simulink model "CartPendsys_continous"  (R2022a)
settings: Solver=VariableStepAuto  StartTime=0.0  StopTime=15  RelTol=1e-3
values from neighbouring files (symbols this model uses):
  Kr = lqr(sysC.A,sysC.B,Q,R)    [sim_pendcart.m]
  Mscale = [eye(4); zeros(2,4)]    [sim_pendcart.m]
  Mscale1 = [eye(3), eye(3)]    [sim_pendcart.m]
  Mscale2 = [eye(2), eye(2)]    [sim_pendcart.m]
  sysC = ss(A,BF,C,[0 0 0 0 0 Vn])    [sim_pendcart.m]
  sysKf = ss(A-Kf*C, [B Kf], eye(4), 0*[B Kf])    [sim_pendcart.m]
  x0 = [1.5 0 pi 0]    [sim_pendcart.m]
settings Model: Creator=samrudh.untgodpr  LastModifiedBy=samrudh.untgodpr
settings DebuggingCC: UnconnectedInputMsg=warning  UnconnectedOutputMsg=warning  UnconnectedLineMsg=warning
settings RTWCC: DLArmComputeVersion=19.05

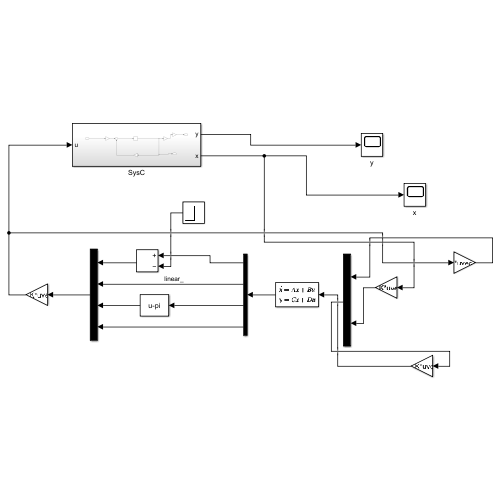
[thumbnail: Simulink's stored preview of the top-level diagram]
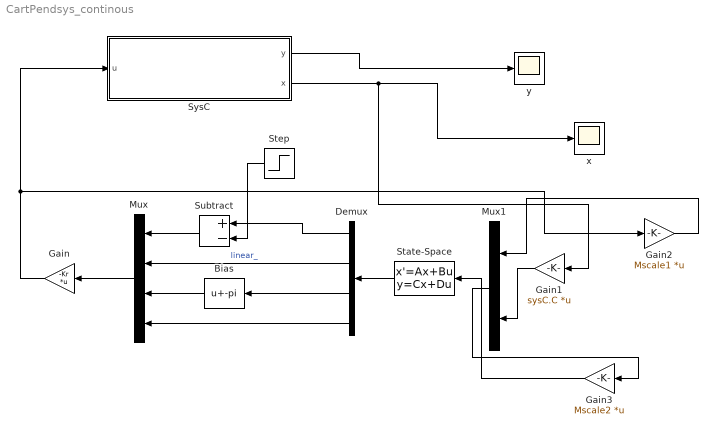
== system CartPendsys_continous ==
  Bias : Bias  Bias=-pi  SaturateOnIntegerOverflow=off
  Demux : Demux
  Gain : Gain  Gain=-Kr  Multiplication=Matrix(K*u) (u vector)
  Gain1 : Gain  Gain=sysC.C  Multiplication=Matrix(K*u) (u vector)
  Gain2 : Gain  Gain=Mscale1  Multiplication=Matrix(K*u) (u vector)
  Gain3 : Gain  Gain=Mscale2  Multiplication=Matrix(K*u) (u vector)
  Mux : Mux
  Mux1 : Mux  Inputs=2
  State-Space : StateSpace  A=sysKf.A  B=sysKf.B  C=sysKf.C  D=sysKf.D  InitialCondition=0
  Step : Step  Time=10  SampleTime=0
  Subtract : Sum  Inputs=+-
  SysC : Subsystem
  x : Scope
  y : Scope
  wires:
  Gain/1 -> Gain2/1, SysC/1(u)
  SysC/1(y) -> y/1
  Mux/1 -> Gain/1
  Demux/1 -> Subtract/1
  Demux/2 -> Mux/2  "linear_"
  Demux/3 -> Bias/1
  Demux/4 -> Mux/4
  Subtract/1 -> Mux/1
  Step/1 -> Subtract/2
  Bias/1 -> Mux/3
  SysC/2(x) -> Gain1/1, x/1
  Gain1/1 -> Mux1/2
  Mux1/1 -> Gain3/1
  State-Space/1 -> Demux/1
  Gain2/1 -> Mux1/1
  Gain3/1 -> State-Space/1

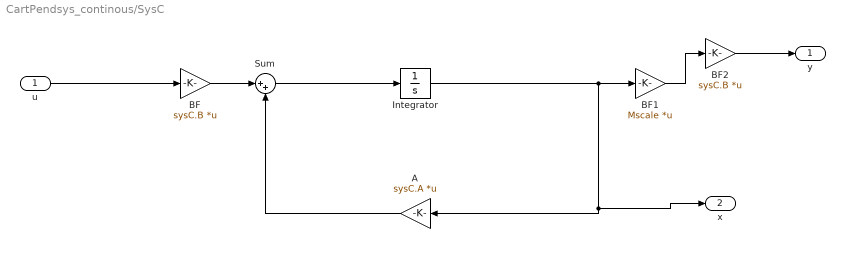
== system CartPendsys_continous/SysC ==
  u : Inport  PortDimensions=6
  A : Gain  Gain=sysC.A  Multiplication=Matrix(K*u)
  BF : Gain  Gain=sysC.B  Multiplication=Matrix(K*u)
  BF1 : Gain  Gain=Mscale  Multiplication=Matrix(K*u)
  BF2 : Gain  Gain=sysC.B  Multiplication=Matrix(K*u) (u vector)
  Integrator : Integrator  InitialCondition=x0
  Sum : Sum  Inputs=|++
  y : Outport
  x : Outport  Port=2
  wires:
  Integrator/1 -> BF1/1, x/1, A/1
  A/1 -> Sum/2
  BF/1 -> Sum/1
  Sum/1 -> Integrator/1
  u/1 -> BF/1
  BF1/1 -> BF2/1
  BF2/1 -> y/1
